simulink model "HPUn_Co"  (R2016b)
settings: configuration reference "CodeGenConfigSet" (kept outside this file)
values from neighbouring files (symbols this model uses):
  HPUn_dvolMeUnMax_C = Calibration.Parameter    [init_HPUn_Co.m]
  HPUn_dvolPmpTolc_CUR = Calibration.Parameter    [init_HPUn_Co.m]
  HPUn_dvolPmpTolc_CURX = Calibration.Parameter    [init_HPUn_Co.m]
  HPUn_etaPmp_MAP = Calibration.Parameter    [init_HPUn_Co.m]
  HPUn_etaPmp_MAPX = Calibration.Parameter    [init_HPUn_Co.m]
  HPUn_etaPmp_MAPY = Calibration.Parameter    [init_HPUn_Co.m]
  HPUn_etaPmpFlTemp_CUR = Calibration.Parameter    [init_HPUn_Co.m]
  HPUn_etaPmpFlTemp_CURX = Calibration.Parameter    [init_HPUn_Co.m]
  HPUn_etaPmpMech_C = Calibration.Parameter    [init_HPUn_Co.m]
  HPUn_nMin_C = Calibration.Parameter    [init_HPUn_Co.m]
  HPUn_rTransCrS_C = Calibration.Parameter    [init_HPUn_Co.m]
  HPUn_volPmp_C = Calibration.Parameter    [init_HPUn_Co.m]
settings Model: Creator=lenovo  LastModifiedBy=wangrui
settings ConfigSetRef: SourceLocation=Base Workspace

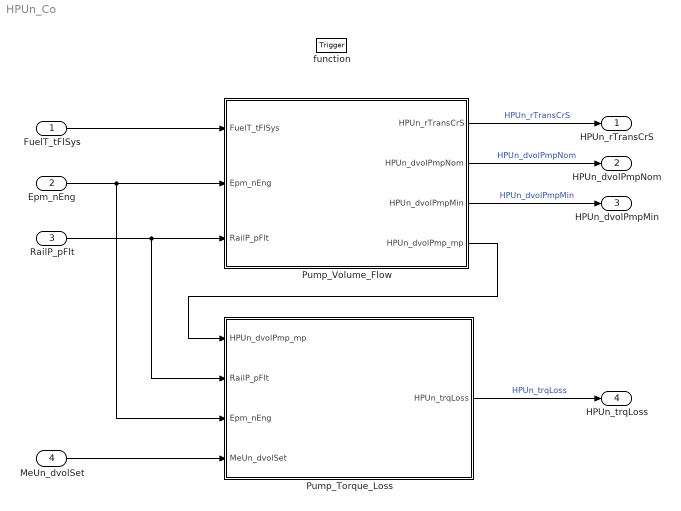
== system HPUn_Co ==
  FuelT_tFlSys : Inport  Tag=deg  Description=Fuel system temperature  OutMin=-50  OutMax=200  OutDataTypeStr=Temp_deg
  Epm_nEng : Inport  Tag=rpm  Description=Engine speed  Port=2  OutMin=0  OutMax=6000  OutDataTypeStr=EngSpeed_rpm
  RailP_pFlt : Inport  Tag=bar  Description=Maximum rail pressure of the last 10 sampling cycle  Port=3  OutMin=0  OutMax=2500  OutDataTypeStr=RailPressure_bar
  MeUn_dvolSet : Inport  Tag=mm^3/s  Description=Setpoint value (volume flow) of rail pressure governing  Port=4  OutMin=-327670  OutMax=327670  OutDataTypeStr=FuelVol_mm3_s
  function : TriggerPort  TriggerType=function-call  VariantControl=Variant
  Pump_Torque_Loss : Subsystem
  "Pump_Volume_Flow " : Subsystem
  HPUn_rTransCrS : Outport  Description=High pressure pump to crankshaft ratio  OutMin=0  OutMax=10  OutDataTypeStr=TransRatio
  HPUn_dvolPmpNom : Outport  Tag=mm^3/s  Description=Pump Nominal value  Port=2  OutMin=0  OutMax=50000  OutDataTypeStr=FuelVol_mm3_s
  HPUn_dvolPmpMin : Outport  Tag=mm^3/s  Description=Minimum pump flow  Port=3  OutMin=0  OutMax=50000  OutDataTypeStr=FuelVol_mm3_s
  HPUn_trqLoss : Outport  Tag=Nm  Description=High pressure pump torque demand  Port=4  OutMin=0  OutMax=1000  OutDataTypeStr=Trq_Nm
  wires:
  MeUn_dvolSet/1 -> Pump_Torque_Loss/4(MeUn_dvolSet)
  Pump_Torque_Loss/1(HPUn_trqLoss) -> HPUn_trqLoss/1  "HPUn_trqLoss"
  Epm_nEng/1 -> "Pump_Volume_Flow "/2(Epm_nEng), Pump_Torque_Loss/3(Epm_nEng)
  RailP_pFlt/1 -> "Pump_Volume_Flow "/3(RailP_pFlt), Pump_Torque_Loss/2(RailP_pFlt)
  FuelT_tFlSys/1 -> "Pump_Volume_Flow "/1(FuelT_tFlSys)
  "Pump_Volume_Flow "/1(HPUn_rTransCrS) -> HPUn_rTransCrS/1  "HPUn_rTransCrS"
  "Pump_Volume_Flow "/2(HPUn_dvolPmpNom) -> HPUn_dvolPmpNom/1  "HPUn_dvolPmpNom"
  "Pump_Volume_Flow "/3(HPUn_dvolPmpMin) -> HPUn_dvolPmpMin/1  "HPUn_dvolPmpMin"
  "Pump_Volume_Flow "/4(HPUn_dvolPmp_mp) -> Pump_Torque_Loss/1(HPUn_dvolPmp_mp)

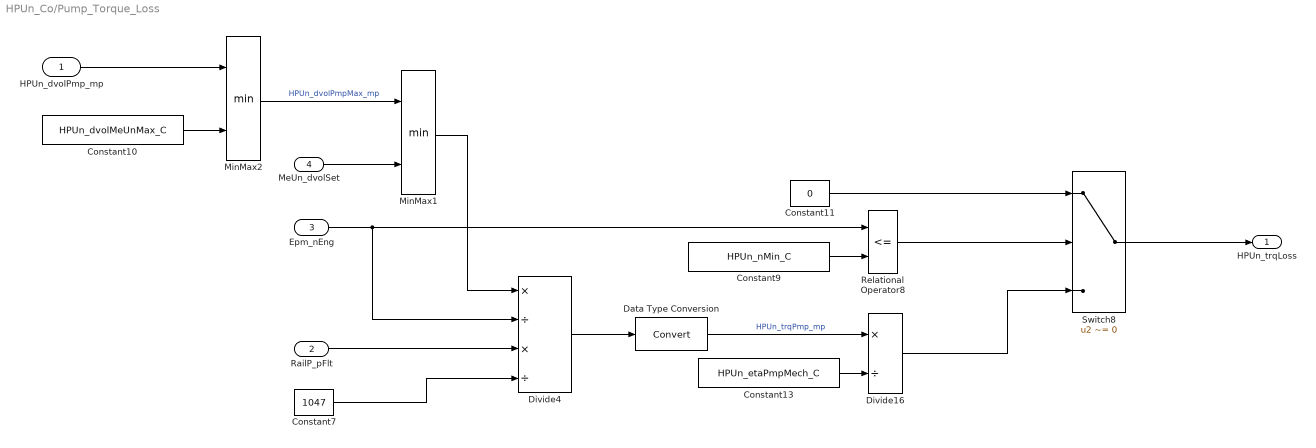
== system HPUn_Co/Pump_Torque_Loss ==
  HPUn_dvolPmp_mp : Inport
  RailP_pFlt : Inport  Port=2
  Epm_nEng : Inport  Port=3
  MeUn_dvolSet : Inport  Tag=mm3/s  Description=Setpoint value (volume flow) of rail pressure governing  Port=4
  Constant10 : Constant  Value=HPUn_dvolMeUnMax_C
  Constant11 : Constant  Value=0  OutDataTypeStr=Inherit: Inherit via back propagation
  Constant13 : Constant  Value=HPUn_etaPmpMech_C
  Constant7 : Constant  Value=1047  OutDataTypeStr=Inherit: Inherit via back propagation
  Constant9 : Constant  Value=HPUn_nMin_C
  Data Type Conversion : DataTypeConversion  RndMeth=Nearest
  Divide16 : Product  RequirementInfo={} %GIDa_9e8150a5_4fde_419b_8aa2_1070a19a8e96  Inputs=*/  OutDataTypeStr=Trq_Nm
  Divide4 : Product  RequirementInfo={'other' 'HPUn_requirements.docx' '@Simulink_requirement_item_17' 'true' '高压油泵扭矩需求' '' } %GIDa_09acea94_7906_48c2_8cb9_17f4726a6ecb  Inputs=*/*/  OutDataTypeStr=fixdt(1,32,7)
  MinMax1 : MinMax  Inputs=2  InputSameDT=on
  MinMax2 : MinMax  Inputs=2  InputSameDT=on
  Relational Operator8 : RelationalOperator  Operator=<=  OutDataTypeStr=boolean  RndMeth=Nearest  InputSameDT=on
  Switch8 : Switch  RequirementInfo={'other' 'HPUn_requirements.docx' '@Simulink_requirement_item_17' 'true' '高压油泵扭矩需求' '' } %GIDa_e0a919f6_6f39_4dd0_bfd8_b66d4e79cff3  Criteria=u2 ~= 0  InputSameDT=on
  HPUn_trqLoss : Outport  Tag=Nm  Description=High pressure pump torque demand
  wires:
  RailP_pFlt/1 -> Divide4/3
  HPUn_dvolPmp_mp/1 -> MinMax2/1
  Epm_nEng/1 -> Divide4/2, Relational Operator8/1
  Constant10/1 -> MinMax2/2
  MinMax2/1 -> MinMax1/1  "HPUn_dvolPmpMax_mp"
  Constant13/1 -> Divide16/2
  Constant7/1 -> Divide4/4
  Data Type Conversion/1 -> Divide16/1  "HPUn_trqPmp_mp"
  Divide4/1 -> Data Type Conversion/1
  MeUn_dvolSet/1 -> MinMax1/2
  MinMax1/1 -> Divide4/1
  Divide16/1 -> Switch8/3
  Switch8/1 -> HPUn_trqLoss/1
  Relational Operator8/1 -> Switch8/2
  Constant11/1 -> Switch8/1
  Constant9/1 -> Relational Operator8/2

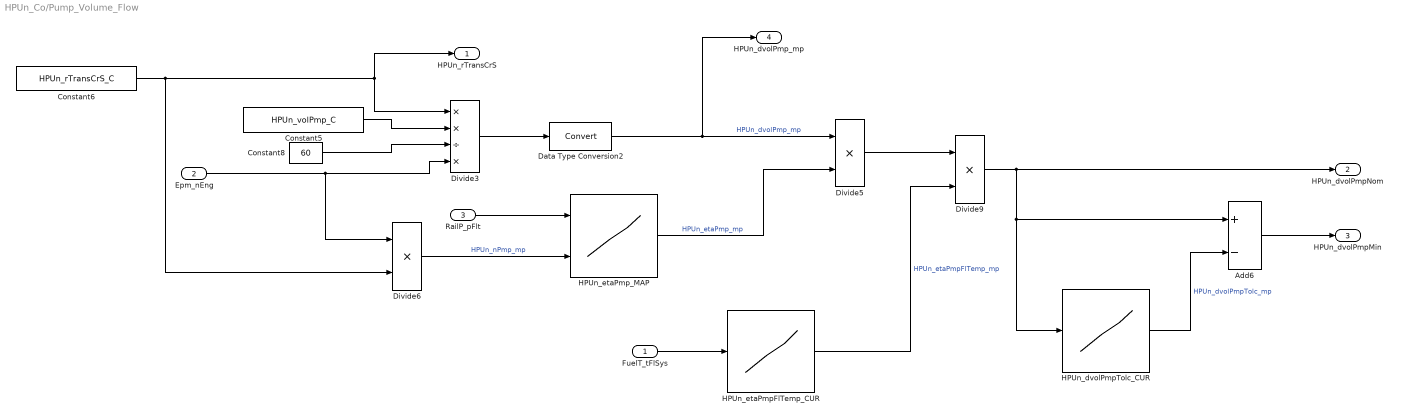
== system HPUn_Co/Pump_Volume_Flow  ==
  FuelT_tFlSys : Inport  Tag=deg  Description=Fuel system temperature
  Epm_nEng : Inport  Tag=rpm  Description=Average engine speed of one cylinder segment  Port=2
  RailP_pFlt : Inport  Tag=bar  Description=Maximum rail pressure of the last 10 ms  Port=3
  Add6 : Sum  RequirementInfo={'other' 'HPUn_requirements.docx' '@Simulink_requirement_item_16' 'true' '高压油泵供油量计算' '' } %GIDa_716e6b58_bc68_4f02_91af_76485cb13d1e  Inputs=+-  InputSameDT=on
  Constant5 : Constant  Value=HPUn_volPmp_C
  Constant6 : Constant  Value=HPUn_rTransCrS_C  SampleTime=-1
  Constant8 : Constant  Value=60  OutDataTypeStr=Inherit: Inherit via back propagation
  Data Type Conversion2 : DataTypeConversion
  Divide3 : Product  RequirementInfo={'other' 'HPUn_requirements.docx' '@Simulink_requirement_item_16' 'true' '高压油泵供油量计算' '' } %GIDa_654690ed_d9c8_4bc2_9609_241520d3be53  Inputs=**/*  OutDataTypeStr=fixdt(1,32,5)
  Divide5 : Product  RequirementInfo={'other' 'HPUn_requirements.docx' '@Simulink_requirement_item_16' 'true' '高压油泵供油量计算' '' } %GIDa_420eff35_dd55_47c0_91de_b3315ceea3b5  Inputs=**  OutDataTypeStr=FuelVol_mm3_s
  Divide6 : Product  RequirementInfo={'other' 'HPUn_requirements.docx' '@Simulink_requirement_item_16' 'true' '高压油泵供油量计算' '' } %GIDa_64df0464_ae49_4cc1_9f1b_62bca5301d1d  Inputs=**  OutDataTypeStr=EngSpeed_rpm
  Divide9 : Product  RequirementInfo={'other' 'HPUn_requirements.docx' '@Simulink_requirement_item_16' 'true' '高压油泵供油量计算' '' } %GIDa_7ee0a1a9_4a41_485b_9f44_37b370de0907  Inputs=**  OutDataTypeStr=FuelVol_mm3_s
  HPUn_dvolPmpTolc_CUR : Lookup_n-D  RequirementInfo={'other' 'HPUn_requirements.docx' '@Simulink_requirement_item_15' 'true' '体积流量调整值查表' '' } %GIDa_b7b90f68_b2b9_4823_9a3b_7dc8c8967f93  NumberOfTableDimensions=1  BreakpointsForDimension1=HPUn_dvolPmpTolc_CURX  BreakpointsForDimension2=HPUn_etaPmp_MAPY  IndexSearchMethod=Linear search  BeginIndexSearchUsingPreviousIndexResult=on  Table=HPUn_dvolPmpTolc_CUR  ExtrapMethod=Clip  UseLastTableValue=on  InternalRulePriority=Speed  OutDataTypeStr=Inherit: Inherit via back propagation  SaturateOnIntegerOverflow=on
  HPUn_etaPmpFlTemp_CUR : Lookup_n-D  RequirementInfo={'other' 'HPUn_requirements.docx' '@Simulink_requirement_item_14' 'true' '基于燃油温度的高压油泵效率查表' '' } %GIDa_e671e765_a093_4421_ba03_cdbf7bf1e7d1  NumberOfTableDimensions=1  BreakpointsForDimension1=HPUn_etaPmpFlTemp_CURX  BreakpointsForDimension2=HPUn_etaPmp_MAPY  IndexSearchMethod=Linear search  BeginIndexSearchUsingPreviousIndexResult=on  Table=HPUn_etaPmpFlTemp_CUR  ExtrapMethod=Clip  UseLastTableValue=on  InternalRulePriority=Speed  OutDataTypeStr=Inherit: Inherit via back propagation  SaturateOnIntegerOverflow=on
  HPUn_etaPmp_MAP : Lookup_n-D  RequirementInfo={'other' 'HPUn_requirements.docx' '@Simulink_requirement_item_13' 'true' '效率查表' '' } %GIDa_6a766265_bce4_4f88_872b_bc238c649675  BreakpointsForDimension1=HPUn_etaPmp_MAPY  BreakpointsForDimension2=HPUn_etaPmp_MAPX  IndexSearchMethod=Linear search  BeginIndexSearchUsingPreviousIndexResult=on  Table=HPUn_etaPmp_MAP  ExtrapMethod=Clip  UseLastTableValue=on  InternalRulePriority=Speed  OutDataTypeStr=Inherit: Inherit via back propagation  SaturateOnIntegerOverflow=on
  HPUn_rTransCrS : Outport  Tag=-  Description=High pressure pump to crankshaft ratio
  HPUn_dvolPmpNom : Outport  Tag=mm3/s  Description=Nominal value  Port=2
  HPUn_dvolPmpMin : Outport  Tag=mm3/s  Description=Minimum pump flow  Port=3
  HPUn_dvolPmp_mp : Outport  Port=4
  wires:
  RailP_pFlt/1 -> HPUn_etaPmp_MAP/1
  Divide9/1 -> HPUn_dvolPmpNom/1, HPUn_dvolPmpTolc_CUR/1, Add6/1
  FuelT_tFlSys/1 -> HPUn_etaPmpFlTemp_CUR/1
  Divide5/1 -> Divide9/1
  HPUn_etaPmp_MAP/1 -> Divide5/2  "HPUn_etaPmp_mp"
  Data Type Conversion2/1 -> HPUn_dvolPmp_mp/1, Divide5/1  "HPUn_dvolPmp_mp"
  Constant8/1 -> Divide3/3
  Divide3/1 -> Data Type Conversion2/1
  Add6/1 -> HPUn_dvolPmpMin/1
  Constant5/1 -> Divide3/2
  Divide6/1 -> HPUn_etaPmp_MAP/2  "HPUn_nPmp_mp"
  HPUn_etaPmpFlTemp_CUR/1 -> Divide9/2  "HPUn_etaPmpFlTemp_mp"
  Epm_nEng/1 -> Divide6/1, Divide3/4
  HPUn_dvolPmpTolc_CUR/1 -> Add6/2  "HPUn_dvolPmpTolc_mp"
  Constant6/1 -> HPUn_rTransCrS/1, Divide3/1, Divide6/2
